simulink model "SimLin"  (R2023a)
settings: Solver=ode45  StartTime=0.0  StopTime=10.0  RelTol=1e-3  EnableMultiTasking=on
values from neighbouring files (symbols this model uses):
  ParamR =     [DataLin.mat]    (also in DataNLin.mat)
settings Model: Creator=nazih  LastModifiedBy=haoyuan
settings SolverCC: AlgebraicLoopSolver=TrustRegion
settings DataIOCC: LimitDataPoints=on  SaveFormat=Array  SignalLoggingSaveFormat=ModelDataLogs  ReturnWorkspaceOutputs=off
settings OptimizationCC: BlockReduction=off  BooleanDataType=off
settings DebuggingCC: SaveWithParameterizedLinksMsg=none  UnderspecifiedInitializationDetection=Classic  MergeDetectMultiDrivingBlocksExec=none  SignalResolutionControl=TryResolveAllWithWarning  MultiTaskDSMMsg=warning  MultiTaskCondExecSysMsg=none  UnconnectedInputMsg=warning  UnconnectedOutputMsg=warning  UnconnectedLineMsg=warning  ArithmeticOperatorsInVariantConditions=warning
settings HardwareCC: TargetUnknown=on
settings ModelReferenceCC: EnableRefExpFcnMdlSchedulingChecks=on  PropagateSignalLabelsOutOfModel=off
settings SFSimCC: SimUseLocalCustomCode=off  CustomCodeUndefinedFunction=UseInterfaceOnly
settings RTWCC: RTWUseLocalCustomCode=off  DLArmComputeVersion=19.05
settings GRTTargetCC: TargetLangStandard=C89/C90 (ANSI)  CombineOutputUpdateFcns=off  GRTInterface=on
settings ConfigComp: CovSaveCumulativeToWorkspaceVar=on  CovSaveSingleToWorkspaceVar=on  CovExternalEMLEnable=off

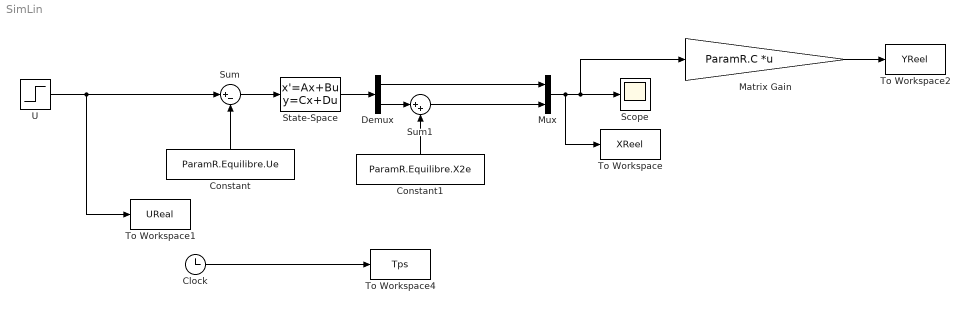
== system SimLin ==
  Clock : Clock
  Constant : Constant  Value=ParamR.Equilibre.Ue
  Constant1 : Constant  Value=ParamR.Equilibre.X2e
  Demux : Demux  Outputs=2
      settings: DisplayOption=none
  Matrix Gain : Gain  Gain=ParamR.C  Multiplication=Matrix(K*u)  SaturateOnIntegerOverflow=on  OutDataTypeStr=Inherit: Same as input  ParamDataTypeStr=Inherit: Same as input
  Mux : Mux  Inputs=2
  Scope : Scope
  State-Space : StateSpace  A=ParamR.A  B=ParamR.B  C=eye(2)  D=zeros(2,1)  InitialCondition=ParamR.X0lin
  Sum : Sum  Inputs=|+-  InputSameDT=on  SaturateOnIntegerOverflow=on  OutDataTypeStr=Inherit: Same as first input
  Sum1 : Sum  Inputs=|++  InputSameDT=on  SaturateOnIntegerOverflow=on  OutDataTypeStr=Inherit: Same as first input
  To Workspace : ToWorkspace  VariableName=XReel  SampleTime=ParamR.Te
  To Workspace1 : ToWorkspace  VariableName=UReal  SampleTime=ParamR.Te
  To Workspace2 : ToWorkspace  VariableName=YReel  SampleTime=ParamR.Te
  To Workspace4 : ToWorkspace  VariableName=Tps  SampleTime=ParamR.Te
  U : Step  Time=4  Before=ParamR.Equilibre.Ue  After=ParamR.Equilibre.Ue+1  SampleTime=0
  wires:
  State-Space/1 -> Demux/1
  U/1 -> Sum/1, To Workspace1/1
  Sum/1 -> State-Space/1
  Constant/1 -> Sum/2
  Demux/2 -> Sum1/1
  Constant1/1 -> Sum1/2
  Sum1/1 -> Mux/2
  Demux/1 -> Mux/1
  Mux/1 -> To Workspace/1, Scope/1, Matrix Gain/1
  Matrix Gain/1 -> To Workspace2/1
  Clock/1 -> To Workspace4/1
